simulink model "Triskar_dynamic_model"  (R2016b)
settings: Solver=ode23t  StartTime=0.0  StopTime=3.0  RelTol=1e-3
values from neighbouring files (symbols this model uses):
  cl = 0    [Kinematic_model_triskar.m]
  cm = 5e-8    (= 5e-08)    [Kinematic_model_triskar.m]
  J = 4.6e-3    (= 0.0046)    [Kinematic_model_triskar.m]    (also in Robot_Parameter.m = 2.125)
  JL = 8e-5    (= 8e-05)    [Kinematic_model_triskar.m]
  Jm = 2.7e-7    (= 2.7e-07)    [Kinematic_model_triskar.m]    (also in Robot_Parameter.m = 3.88e-07)
  Ke = 0.0145    [Kinematic_model_triskar.m]
  Klr = 1/8.71    (= 0.114810562572)    [Kinematic_model_triskar.m]
  Km = 0.0144    [Kinematic_model_triskar.m]
  L = 7e-2    (= 0.07)    [Kinematic_model_triskar.m]    (also in Robot_Parameter.m = 0.00011)
  m = 2.36    [Kinematic_model_triskar.m]
  n = 14    [Kinematic_model_triskar.m]
  r = 2e-2    (= 0.02)    [Kinematic_model_triskar.m]
settings Model: Creator=davide  LastModifiedBy=davide

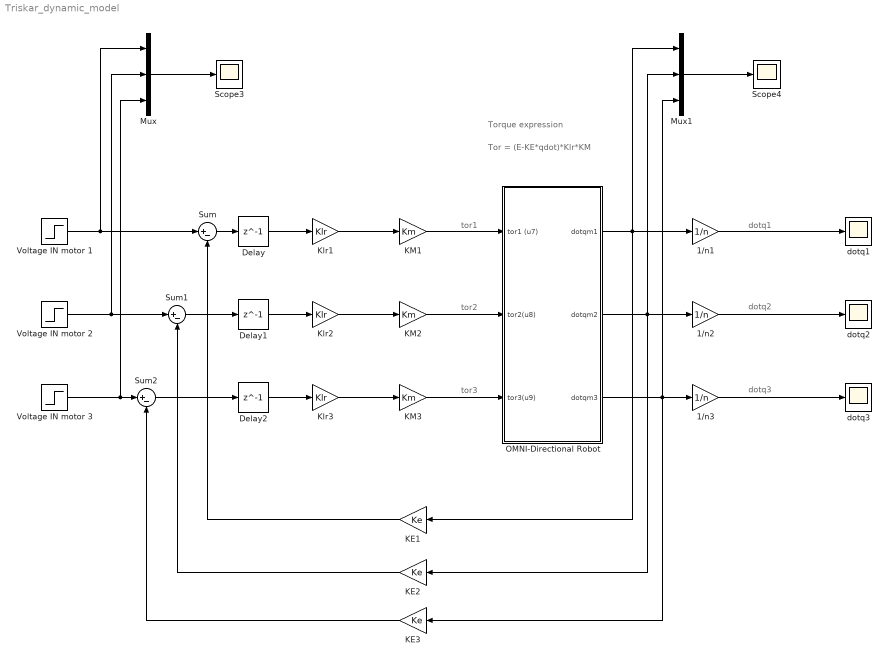
== system Triskar_dynamic_model ==
  note: dotq3
  note: dotq2
  note: dotq1
  note: tor3
  note: tor2
  note: tor1
  note: Torque expression
  note: Tor = (E-KE*qdot)*Klr*KM
  1/n1 : Gain  Gain=1/n
  1/n2 : Gain  Gain=1/n
  1/n3 : Gain  Gain=1/n
  Delay : Delay  DelayLength=1  InitialCondition=0
  Delay1 : Delay  DelayLength=1  InitialCondition=0
  Delay2 : Delay  DelayLength=1  InitialCondition=0
  KE1 : Gain  Gain=Ke
  KE2 : Gain  Gain=Ke
  KE3 : Gain  Gain=Ke
  KM1 : Gain  Gain=Km
  KM2 : Gain  Gain=Km
  KM3 : Gain  Gain=Km
  Klr1 : Gain  Gain=Klr
  Klr2 : Gain  Gain=Klr
  Klr3 : Gain  Gain=Klr
  Mux : Mux  Inputs=3
  Mux1 : Mux  Inputs=3
  OMNI-Directional Robot : Subsystem
  Scope3 : Scope
  Scope4 : Scope
  Sum : Sum  Inputs=|+-
  Sum1 : Sum  Inputs=|+-
  Sum2 : Sum  Inputs=|+-
  Voltage IN motor 1 : Step  After=12  SampleTime=0
  Voltage IN motor 2 : Step  After=12  SampleTime=0
  Voltage IN motor 3 : Step  After=12  SampleTime=0
  dotq1 : Scope
  dotq2 : Scope
  dotq3 : Scope
  wires:
  Voltage IN motor 3/1 -> Mux/3, Sum2/1
  Voltage IN motor 2/1 -> Mux/2, Sum1/1
  Voltage IN motor 1/1 -> Mux/1, Sum/1
  Klr1/1 -> KM1/1
  KM1/1 -> OMNI-Directional Robot/1(tor1 (u7))
  Klr2/1 -> KM2/1
  KM2/1 -> OMNI-Directional Robot/2(tor2(u8))
  Klr3/1 -> KM3/1
  KM3/1 -> OMNI-Directional Robot/3(tor3(u9))
  OMNI-Directional Robot/3(dotqm3) -> Mux1/3, KE3/1, 1/n3/1
  OMNI-Directional Robot/2(dotqm2) -> Mux1/2, KE2/1, 1/n2/1
  OMNI-Directional Robot/1(dotqm1) -> Mux1/1, KE1/1, 1/n1/1
  KE1/1 -> Sum/2
  KE2/1 -> Sum1/2
  KE3/1 -> Sum2/2
  Sum/1 -> Delay/1
  Delay/1 -> Klr1/1
  Sum1/1 -> Delay1/1
  Delay1/1 -> Klr2/1
  Sum2/1 -> Delay2/1
  Delay2/1 -> Klr3/1
  1/n1/1 -> dotq1/1
  1/n2/1 -> dotq2/1
  1/n3/1 -> dotq3/1
  Mux/1 -> Scope3/1
  Mux1/1 -> Scope4/1

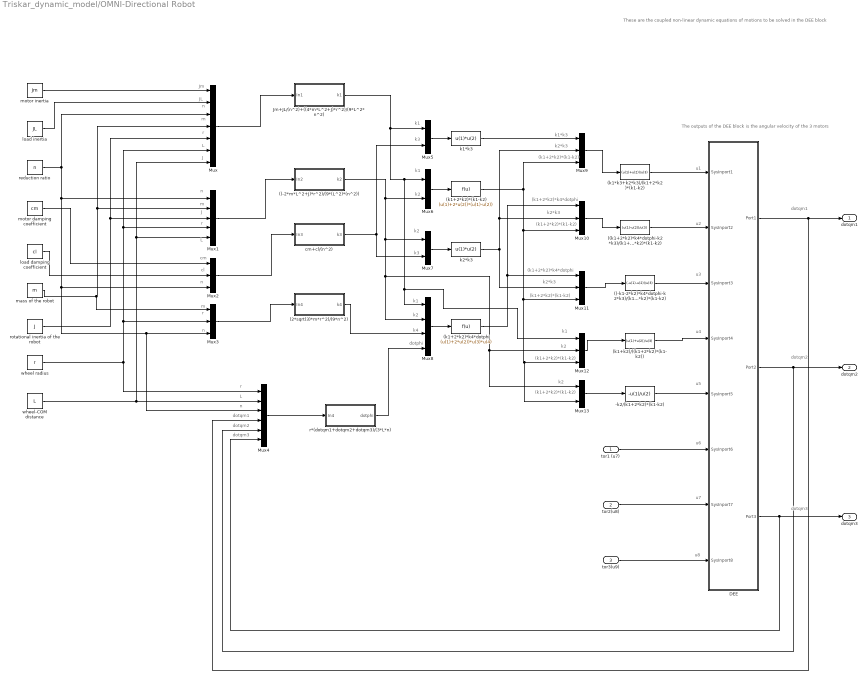
== system Triskar_dynamic_model/OMNI-Directional Robot ==
  note: (k1+2*k2)*(k1-k2)
  note: k2
  note: (k1+2*k2)*(k1-k2)
  note: k2
  note: k1
  note: (k1+2*k2)*(k1-k2)
  note: k2*k3
  note: (k1+2*k2)*k4*dotphi
  note: (k1+2*k2)*(k1-k2)
  note: k2*k3
  note: (k1+2*k2)*k4*dotphi
  note: (k1+2*k2)*(k1-k2)
  note: k2*k3
  note: k1*k3
  note: dotphi
  note: k4
  note: k2
  note: k1
  note: k3
  note: k2
  note: k2
  note: k1
  note: k3
  note: k1
  note: The outputs of the DEE block is the angular velocity of the 3 motors
  note: These are the coupled non-linear dynamic equations of motions to be solved in the DEE block
  note: u8
  note: u7
  note: u6
  note: u5
  note: u4
  note: u3
  note: u2
  note: u1
  note: dotqm3
  note: dotqm2
  note: dotqm1
  note: dotqm3
  note: dotqm2
  note: dotqm1
  note: n
  note: L
  note: r
  note: n
  note: r
  note: m
  note: n
  note: cl
  note: cm
  note: L
  note: r
  note: J
  note: m
  note: n
  note: J
  note: L
  note: r
  note: m
  note: n
  note: JL
  note: Jm
  tor1 (u7) : Inport
  tor2(u8) : Inport  Port=2
  tor3(u9) : Inport  Port=3
  ((-2*m*L^2+J)*r^2)/(9*(L^2)*(n^2)) : Subsystem
  ((-k1-2*k2)*k4*dotphi-k2*k3)/(k1+2*k2)*(k1-k2) : Fcn  Expr=(-u(1)-u(2))/u(3)
  ((k1+2*k2)*k4*dotphi-k2*k3)/(k1+2*k2)*(k1-k2) : Fcn  Expr=(u(1)-u(2))/u(3)
  (2*sqrt(3)*m*r^2)/(9*n^2) : Subsystem
  (k1*k3+k2*k3)/(k1+2*k2)*(k1-k2) : Fcn  Expr=(u(1)+u(2))/u(3)
  (k1+2*k2)*(k1-k2) : Fcn  Expr=(u(1)+2*u(2))*(u(1)-u(2))
  (k1+2*k2)*k4*dotphi : Fcn  Expr=(u(1)+2*u(2))*u(3)*u(4)
  (k1+k2)/((k1+2*k2)*(k1-k2)) : Fcn  Expr=(u(1)+u(2))/u(3)
  -k2/(k1+2*k2)*(k1-k2) : Fcn  Expr=-u(1)/u(2)
  DEE : Subsystem  mask(Differential Equation Editor (DEE)){}
      settings: OpenFcn=diffeqed
      mask Display: disp('ROBOT')
  Jm+JL/(n^2)+((4*m*L^2+J)*r^2)/(9*L^2*n^2) : Subsystem
  Mux : Mux  Inputs=7
  Mux1 : Mux  Inputs=5
  Mux{2..3,9..12} (6 alike) : Mux  Inputs=3
  Mux{5..7,13} (4 alike) : Mux  Inputs=2
  Mux4 : Mux  Inputs=6
  Mux8 : Mux
  cm+cl/(n^2) : Subsystem
  k1*k3 : Fcn  Expr=u(1)*u(2)
  k2*k3 : Fcn  Expr=u(1)*u(2)
  load damping coefficient : Constant  Value=cl
  load inertia : Constant  Value=JL
  mass of the robot : Constant  Value=m
  motor damping coefficient : Constant  Value=cm
  motor inertia : Constant  Value=Jm
  r*(dotqm1+dotqm2+dotqm3)/(3*L*n) : Subsystem
  reduction ratio : Constant  Value=n
  rotational inertia of the robot : Constant  Value=J
  wheel radius : Constant  Value=r
  wheel-COM distance : Constant  Value=L
  dotqm1 : Outport
  dotqm2 : Outport  Port=2
  dotqm3 : Outport  Port=3
  wires:
  motor inertia/1 -> Mux/1
  load inertia/1 -> Mux/2
  reduction ratio/1 -> Mux/3, Mux4/3, Mux3/3, Mux2/3, Mux1/1
  mass of the robot/1 -> Mux3/1, Mux1/2, Mux/4
  rotational inertia of the robot/1 -> Mux1/3, Mux/5
  wheel radius/1 -> Mux4/1, Mux3/2, Mux1/4, Mux/6
  wheel-COM distance/1 -> Mux4/2, Mux1/5, Mux/7
  motor damping coefficient/1 -> Mux2/1
  load damping coefficient/1 -> Mux2/2
  Mux/1 -> Jm+JL/(n^2)+((4*m*L^2+J)*r^2)/(9*L^2*n^2)/1(In1)
  Mux1/1 -> ((-2*m*L^2+J)*r^2)/(9*(L^2)*(n^2))/1(In2)
  Mux2/1 -> cm+cl/(n^2)/1(In3)
  Mux3/1 -> (2*sqrt(3)*m*r^2)/(9*n^2)/1(In4)
  Mux4/1 -> r*(dotqm1+dotqm2+dotqm3)/(3*L*n)/1(In4)
  Mux5/1 -> k1*k3/1
  Mux6/1 -> (k1+2*k2)*(k1-k2)/1
  Mux7/1 -> k2*k3/1
  r*(dotqm1+dotqm2+dotqm3)/(3*L*n)/1(dotphi) -> Mux8/4
  cm+cl/(n^2)/1(k3) -> Mux7/2, Mux5/2
  ((-2*m*L^2+J)*r^2)/(9*(L^2)*(n^2))/1(k2) -> Mux6/2, Mux13/1, Mux12/2, Mux8/2, Mux7/1
  (2*sqrt(3)*m*r^2)/(9*n^2)/1(k4) -> Mux8/3
  Mux8/1 -> (k1+2*k2)*k4*dotphi/1
  k1*k3/1 -> Mux9/1
  k2*k3/1 -> Mux11/2, Mux10/2, Mux9/2
  (k1+2*k2)*(k1-k2)/1 -> Mux13/2, Mux12/3, Mux11/3, Mux10/3, Mux9/3
  (k1+2*k2)*k4*dotphi/1 -> Mux11/1, Mux10/1
  Jm+JL/(n^2)+((4*m*L^2+J)*r^2)/(9*L^2*n^2)/1(k1) -> Mux12/1, Mux8/1, Mux6/1, Mux5/1
  tor3(u9)/1 -> DEE/8(SysInport8)
  tor2(u8)/1 -> DEE/7(SysInport7)
  tor1 (u7)/1 -> DEE/6(SysInport6)
  Mux9/1 -> (k1*k3+k2*k3)/(k1+2*k2)*(k1-k2)/1
  (k1*k3+k2*k3)/(k1+2*k2)*(k1-k2)/1 -> DEE/1(SysInport1)
  Mux10/1 -> ((k1+2*k2)*k4*dotphi-k2*k3)/(k1+2*k2)*(k1-k2)/1
  ((k1+2*k2)*k4*dotphi-k2*k3)/(k1+2*k2)*(k1-k2)/1 -> DEE/2(SysInport2)
  Mux11/1 -> ((-k1-2*k2)*k4*dotphi-k2*k3)/(k1+2*k2)*(k1-k2)/1
  ((-k1-2*k2)*k4*dotphi-k2*k3)/(k1+2*k2)*(k1-k2)/1 -> DEE/3(SysInport3)
  Mux12/1 -> (k1+k2)/((k1+2*k2)*(k1-k2))/1
  (k1+k2)/((k1+2*k2)*(k1-k2))/1 -> DEE/4(SysInport4)
  Mux13/1 -> -k2/(k1+2*k2)*(k1-k2)/1
  -k2/(k1+2*k2)*(k1-k2)/1 -> DEE/5(SysInport5)
  DEE/3(Port3) -> Mux4/6, dotqm3/1
  DEE/2(Port2) -> Mux4/5, dotqm2/1
  DEE/1(Port1) -> dotqm1/1, Mux4/4

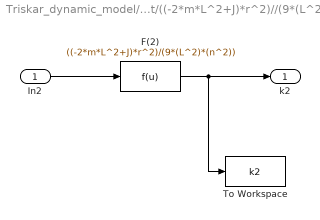
== system Triskar_dynamic_model/OMNI-Directional Robot/((-2*m*L^2+J)*r^2)//(9*(L^2)*(n^2)) ==
  In2 : Inport
  F(2) : Fcn  Expr=((-2*m*L^2+J)*r^2)/(9*(L^2)*(n^2))
  To Workspace : ToWorkspace  VariableName=k2  SampleTime=-1
      settings: MaxDataPoints=1  Save2DSignal=2-D array (concatenate along first dimension)
  k2 : Outport
  wires:
  In2/1 -> F(2)/1
  F(2)/1 -> To Workspace/1, k2/1

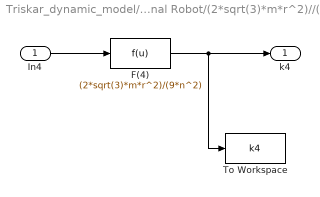
== system Triskar_dynamic_model/OMNI-Directional Robot/(2*sqrt(3)*m*r^2)//(9*n^2) ==
  In4 : Inport
  F(4) : Fcn  Expr=(2*sqrt(3)*m*r^2)/(9*n^2)
  To Workspace : ToWorkspace  VariableName=k4  SampleTime=-1
      settings: MaxDataPoints=1  Save2DSignal=2-D array (concatenate along first dimension)
  k4 : Outport
  wires:
  F(4)/1 -> To Workspace/1, k4/1
  In4/1 -> F(4)/1

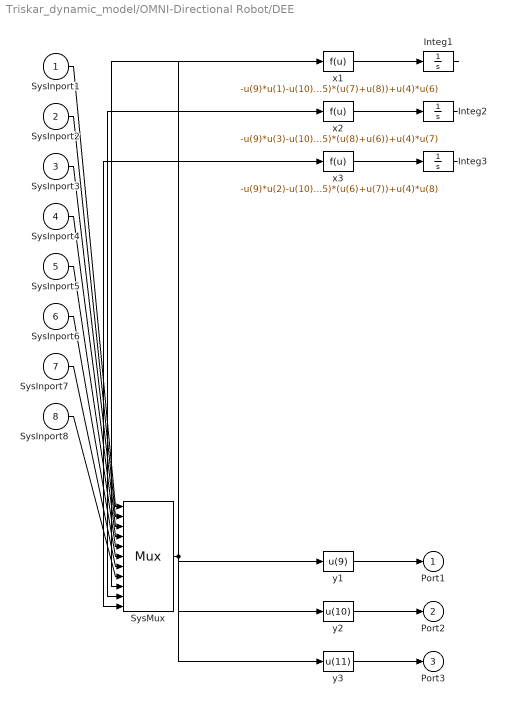
== system Triskar_dynamic_model/OMNI-Directional Robot/DEE ==
  SysInport1 : Inport
  SysInport2 : Inport  Port=2
  SysInport3 : Inport  Port=3
  SysInport4 : Inport  Port=4
  SysInport5 : Inport  Port=5
  SysInport6 : Inport  Port=6
  SysInport7 : Inport  Port=7
  SysInport8 : Inport  Port=8
  Integ1 : Integrator
  Integ2 : Integrator
  Integ3 : Integrator
  SysMux : Mux  Inputs=11
  x1 : Fcn  Expr=-u(9)*u(1)-u(10)*u(2)-u(11)*u(3)+u(5)*(u(7)+u(8))+u(4)*u(6)
  x2 : Fcn  Expr=-u(9)*u(3)-u(10)*u(1)-u(11)*u(2)+u(5)*(u(8)+u(6))+u(4)*u(7)
  x3 : Fcn  Expr=-u(9)*u(2)-u(10)*u(3)-u(11)*u(1)+u(5)*(u(6)+u(7))+u(4)*u(8)
  y1 : Fcn  Expr=u(9)
  y2 : Fcn  Expr=u(10)
  y3 : Fcn  Expr=u(11)
  Port1 : Outport
  Port2 : Outport  Port=2
  Port3 : Outport  Port=3
  wires:
  SysInport1/1 -> SysMux/1
  SysInport2/1 -> SysMux/2
  SysInport3/1 -> SysMux/3
  SysInport4/1 -> SysMux/4
  SysInport5/1 -> SysMux/5
  SysInport6/1 -> SysMux/6
  SysInport7/1 -> SysMux/7
  SysInport8/1 -> SysMux/8
  SysMux/1 -> x1/1, x2/1, x3/1, y1/1, y2/1, y3/1
  x1/1 -> Integ1/1
  Integ1/1 -> SysMux/9
  x2/1 -> Integ2/1
  Integ2/1 -> SysMux/10
  x3/1 -> Integ3/1
  Integ3/1 -> SysMux/11
  y1/1 -> Port1/1
  y2/1 -> Port2/1
  y3/1 -> Port3/1

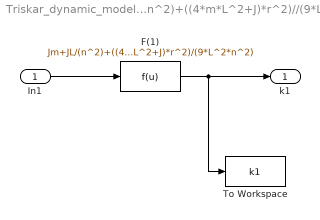
== system Triskar_dynamic_model/OMNI-Directional Robot/Jm+JL//(n^2)+((4*m*L^2+J)*r^2)//(9*L^2*n^2) ==
  In1 : Inport
  F(1) : Fcn  Expr=Jm+JL/(n^2)+((4*m*L^2+J)*r^2)/(9*L^2*n^2)
  To Workspace : ToWorkspace  VariableName=k1  SampleTime=-1
      settings: MaxDataPoints=1  Save2DSignal=2-D array (concatenate along first dimension)
  k1 : Outport
  wires:
  In1/1 -> F(1)/1
  F(1)/1 -> To Workspace/1, k1/1

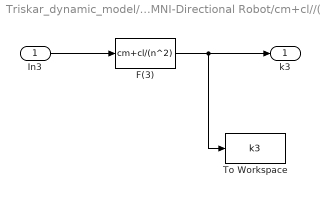
== system Triskar_dynamic_model/OMNI-Directional Robot/cm+cl//(n^2) ==
  In3 : Inport
  F(3) : Fcn  Expr=cm+cl/(n^2)
  To Workspace : ToWorkspace  VariableName=k3  SampleTime=-1
      settings: MaxDataPoints=1  Save2DSignal=2-D array (concatenate along first dimension)
  k3 : Outport
  wires:
  F(3)/1 -> To Workspace/1, k3/1
  In3/1 -> F(3)/1

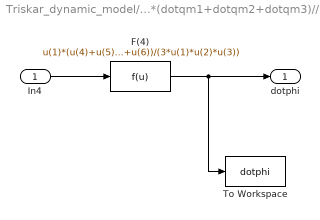
== system Triskar_dynamic_model/OMNI-Directional Robot/r*(dotqm1+dotqm2+dotqm3)//(3*L*n) ==
  In4 : Inport
  F(4) : Fcn  Expr=u(1)*(u(4)+u(5)+u(6))/(3*u(1)*u(2)*u(3))
  To Workspace : ToWorkspace  VariableName=dotphi  SampleTime=-1
      settings: MaxDataPoints=1  Save2DSignal=2-D array (concatenate along first dimension)
  dotphi : Outport
  wires:
  F(4)/1 -> To Workspace/1, dotphi/1
  In4/1 -> F(4)/1
